simulink model "Version_Nov_21"  (R2022a)
settings: Solver=FixedStepAuto  StartTime=0.0  StopTime=60  FixedStep=1e-3  RelTol=1e-3  EnableMultiTasking=on
undefined symbols (not defined in the file): D10, D11, D12, D13, D2, D3, D4, D5, D6, D7, D8, D9, PTA0, PTA1, PTA2, PTB23, PTB9, PTC2, PTC3, PTC4, PTD0, PTD1, PTD2, PTD3
libraries: frdmk64flib x13
settings Model: ExtModeTrigDuration=5  Creator=ethan  LastModifiedBy=ethan
settings OptimizationCC: EnhancedBackFolding=on  PassReuseOutputArgsAs=Individual arguments  ZeroExternalMemoryAtStartup=off  ZeroInternalMemoryAtStartup=off  MaxStackSize=64  OptimizeBlockOrder=speed  DifferentSizesBufferReuse=on  OptimizationCustomize=off  EfficientTunableParamExpr=on
settings DebuggingCC: ParameterTunabilityLossMsg=error
settings HardwareCC: ProdBitPerPointer=32  ProdBitPerSizeT=32  ProdBitPerPtrDiffT=32  ProdLargestAtomicInteger=Long  ProdLargestAtomicFloat=Double  ProdWordSize=32  ProdHWDeviceType=ARM Compatible->ARM Cortex
settings SFSimCC: MATLABDynamicMemAlloc=off
settings RTWCC: SystemTargetFile=ert.tlc  HardwareBoard=NXP FRDM-K64F  TLCOptions="-aInlineSetEventsForThisBaseRateFcn=TLC_FALSE -aSuppressMultiTaskScheduler=TLC_FALSE  -aRateBasedStepFcn=0"  TemplateMakefile=ert_default_tmf  Toolchain=GNU Tools for ARM Embedded Processors
settings CodeAppCC: ForceParamTrailComments=on  IgnoreCustomStorageClasses=off  OperatorAnnotations=on  SimulinkDataObjDesc=on  SFDataObjDesc=on  InsertBlockDesc=on
settings ERTTargetCC: ExtModeTransport=4  ExtModeMexFile=sendToCommService

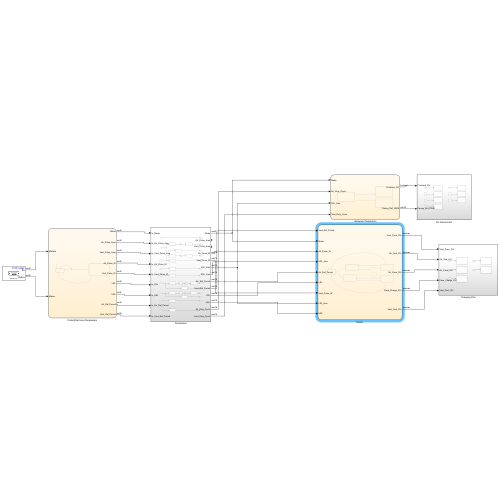
[thumbnail: Simulink's stored preview of the top-level diagram]
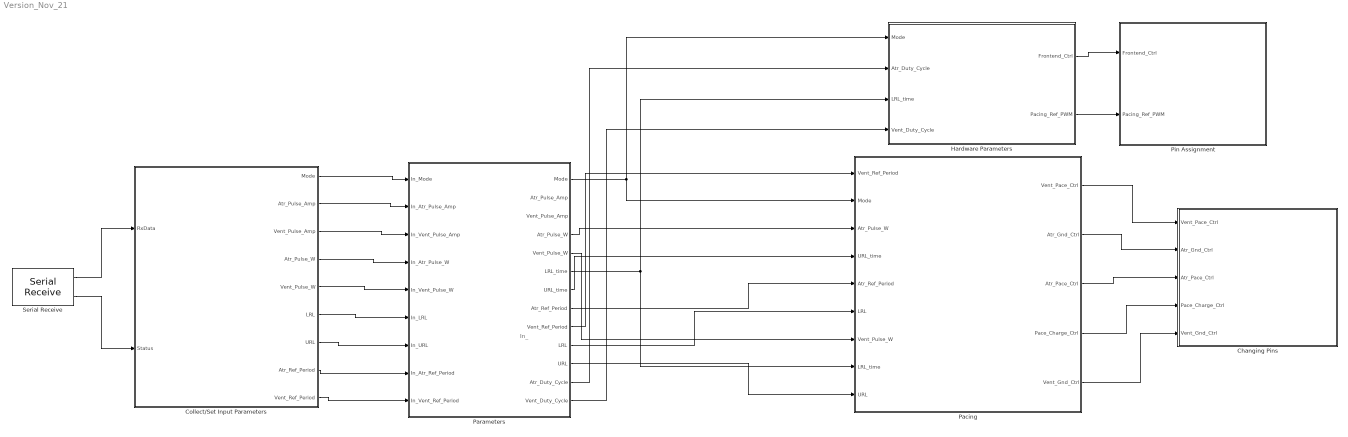
== system Version_Nov_21 ==
  note: In_
  Changing Pins : Subsystem
  Collect/Set Input Parameters : Stateflow chart  TreatAsAtomicUnit=on
      settings: PortSchema="{\"entries\":[{\"content\":{\"sides\":[{\"content\":{\"connectorIds\":[\"In1\",\"In2\"]},\"type\":\"ConnectorPlacement.EquallySpacedRectSide\",\"uuid\":\"dc51e4f5-5341-418f-80a9-38d3dc8e9b6e\"},{\"content\":{\"connectorIds\":[\"Out1\",\"Out3\",\"Out6\",\"Out2\",\"Out7\",\"Out9\",\"Out5\",\"Out4\",\"Out8\"],\"side\":\"RIGHT\"},\"type\":\"ConnectorPlacement.EquallySpacedRectSide\",\"uuid\":\"313c6298-b0b7-4ff0-85ba-dbaa1c18177a\"},{\"content\":{\"connectorIds\":[],\"side\":\"TOP\"},\"type\":\"ConnectorPlacement.EquallySpacedRectSide\",\"uuid\":\"6f377806-6de9-4b84-8111-50855010f7f2\"}]},\"type\":\"ConnectorPlacement.EquallySpacedConnector\",\"uuid\":\"8b0403f6-9322-46f9-82a4-778a28822a3d\"}],\"packageUris\":[\"http://schema.mathworks.com/mf0/Connector/R2020b\"],\"version\":\"1.0\"}"
  Hardware Parameters : Stateflow chart  TreatAsAtomicUnit=on
  Pacing : Stateflow chart  TreatAsAtomicUnit=on
      settings: PortSchema="{\"entries\":[{\"content\":{\"sides\":[{\"content\":{\"connectorIds\":[\"In9\",\"In1\",\"In3\",\"In6\",\"In7\",\"In8\",\"In4\",\"In5\",\"In2\"]},\"type\":\"ConnectorPlacement.EquallySpacedRectSide\",\"uuid\":\"cbd26b3d-27cb-4744-9a6d-2e29f16e2c2e\"},{\"content\":{\"connectorIds\":[\"Out1\",\"Out2\",\"Out3\",\"Out4\",\"Out5\"],\"side\":\"RIGHT\"},\"type\":\"ConnectorPlacement.EquallySpacedRectSide\",\"uuid\":\"25c89074-e17e-4898-a31a-c42a3e343a2e\"},{\"content\":{\"connectorIds\":[],\"side\":\"TOP\"},\"type\":\"ConnectorPlacement.EquallySpacedRectSide\",\"uuid\":\"e4014b57-3770-4bf4-bd9b-5c9114757f0a\"}]},\"type\":\"ConnectorPlacement.EquallySpacedConnector\",\"uuid\":\"9ef350bf-8d26-4971-b7d1-0d0774d6b5a5\"}],\"packageUris\":[\"http://schema.mathworks.com/mf0/Connector/R2020b\"],\"version\":\"1.0\"}"
  Parameters : Subsystem
  Pin Assignment : Subsystem
  Serial Receive : frdmk64flib/Serial Receive  SCIModule=0  Baudrate=uint32(9600)  Parity=None  StopBits=1  HardwareFlowControl=None  ByteOrder=LittleEndian  DataType=uint8  DataLength=10  BlockingMode=off  OutputStatus=on  SampleTime=-1
  wires:
  Serial Receive/1 -> Collect/Set Input Parameters/1(RxData)
  Serial Receive/2 -> Collect/Set Input Parameters/2(Status)
  Collect/Set Input Parameters/1(Mode) -> Parameters/1(In_Mode)
  Collect/Set Input Parameters/3(Atr_Pulse_Amp) -> Parameters/2(In_Atr_Pulse_Amp)
  Collect/Set Input Parameters/6(Vent_Pulse_Amp) -> Parameters/3(In_Vent_Pulse_Amp)
  Collect/Set Input Parameters/4(Atr_Ref_Period) -> Parameters/8(In_Atr_Ref_Period)
  Collect/Set Input Parameters/5(URL) -> Parameters/7(In_URL)
  Collect/Set Input Parameters/9(LRL) -> Parameters/6(In_LRL)
  Collect/Set Input Parameters/8(Vent_Ref_Period) -> Parameters/9(In_Vent_Ref_Period)
  Collect/Set Input Parameters/2(Atr_Pulse_W) -> Parameters/4(In_Atr_Pulse_W)
  Pacing/1(Vent_Pace_Ctrl) -> Changing Pins/1(Vent_Pace_Ctrl)
  Pacing/2(Atr_Gnd_Ctrl) -> Changing Pins/2(Atr_Gnd_Ctrl)
  Pacing/3(Atr_Pace_Ctrl) -> Changing Pins/3(Atr_Pace_Ctrl)
  Pacing/4(Pace_Charge_Ctrl) -> Changing Pins/4(Pace_Charge_Ctrl)
  Pacing/5(Vent_Gnd_Ctrl) -> Changing Pins/5(Vent_Gnd_Ctrl)
  Collect/Set Input Parameters/7(Vent_Pulse_W) -> Parameters/5(In_Vent_Pulse_W)
  Parameters/1(Mode) -> Hardware Parameters/1(Mode), Pacing/1(Mode)
  Parameters/4(Atr_Pulse_W) -> Pacing/3(Atr_Pulse_W)
  Parameters/5(Vent_Pulse_W) -> Pacing/4(Vent_Pulse_W)
  Parameters/6(LRL_time) -> Hardware Parameters/3(LRL_time), Pacing/5(LRL_time)
  Parameters/7(URL_time) -> Pacing/6(URL_time)
  Parameters/8(Atr_Ref_Period) -> Pacing/7(Atr_Ref_Period)
  Parameters/9(Vent_Ref_Period) -> Pacing/9(Vent_Ref_Period)
  Parameters/10(LRL) -> Pacing/8(LRL)
  Parameters/11(URL) -> Pacing/2(URL)
  Parameters/12(Atr_Duty_Cycle) -> Hardware Parameters/2(Atr_Duty_Cycle)
  Parameters/13(Vent_Duty_Cycle) -> Hardware Parameters/4(Vent_Duty_Cycle)
  Hardware Parameters/1(Frontend_Ctrl) -> Pin Assignment/1(Frontend_Ctrl)
  Hardware Parameters/2(Pacing_Ref_PWM) -> Pin Assignment/2(Pacing_Ref_PWM)

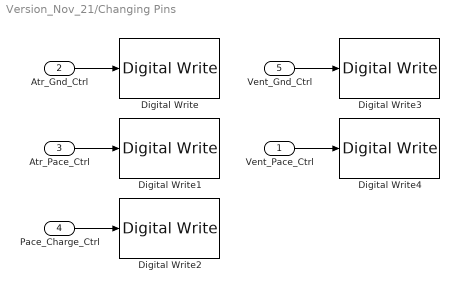
== system Version_Nov_21/Changing Pins ==
  Vent_Pace_Ctrl : Inport
  Atr_Gnd_Ctrl : Inport  Port=2
  Atr_Pace_Ctrl : Inport  Port=3
  Pace_Charge_Ctrl : Inport  Port=4
  Vent_Gnd_Ctrl : Inport  Port=5
  Digital Write : frdmk64flib/Digital Write  Whichpin=PTD2 (D11)
  Digital Write1 : frdmk64flib/Digital Write  Whichpin=PTA0 (D8)
  Digital Write2 : frdmk64flib/Digital Write  Whichpin=PTB9 (D2)
  Digital Write3 : frdmk64flib/Digital Write  Whichpin=PTD3 (D12)
  Digital Write4 : frdmk64flib/Digital Write  Whichpin=PTC4 (D9)
  wires:
  Atr_Gnd_Ctrl/1 -> Digital Write/1
  Atr_Pace_Ctrl/1 -> Digital Write1/1
  Pace_Charge_Ctrl/1 -> Digital Write2/1
  Vent_Gnd_Ctrl/1 -> Digital Write3/1
  Vent_Pace_Ctrl/1 -> Digital Write4/1

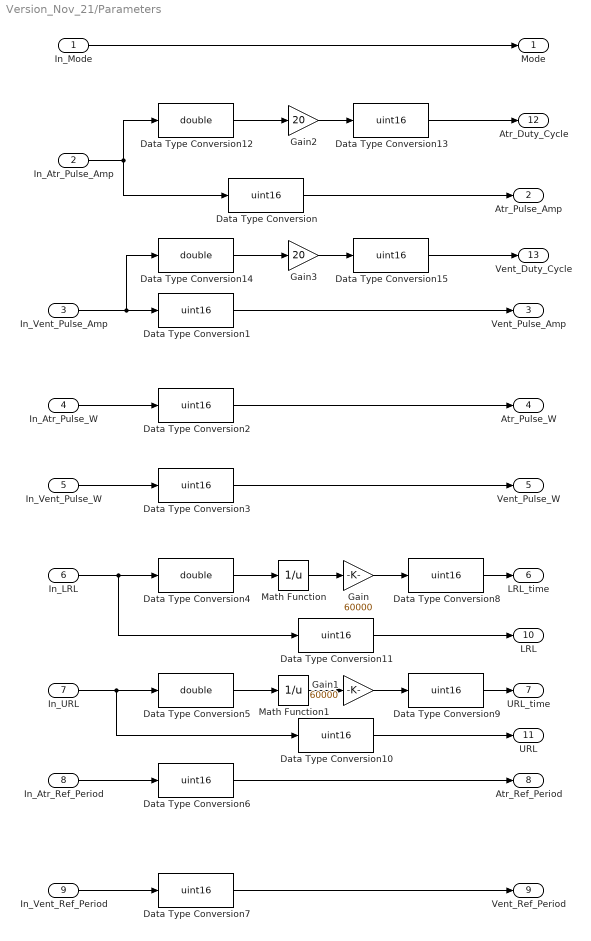
== system Version_Nov_21/Parameters ==
  In_Mode : Inport
  In_Atr_Pulse_Amp : Inport  Port=2
  In_Vent_Pulse_Amp : Inport  Port=3
  In_Atr_Pulse_W : Inport  Port=4
  In_Vent_Pulse_W : Inport  Port=5
  In_LRL : Inport  Port=6
  In_URL : Inport  Port=7
  In_Atr_Ref_Period : Inport  Port=8
  In_Vent_Ref_Period : Inport  Port=9
  Data Type Conversion{,1..3,6..11,13,15} (12 alike) : DataTypeConversion  OutDataTypeStr=uint16  SaturateOnIntegerOverflow=off  RndMeth=Floor
  Data Type Conversion{4..5,12,14} (4 alike) : DataTypeConversion  OutDataTypeStr=double  SaturateOnIntegerOverflow=off  RndMeth=Floor
  Gain : Gain  Gain=60000
  Gain1 : Gain  Gain=60000
  Gain2 : Gain  Gain=20
  Gain3 : Gain  Gain=20
  Math Function : Math  Operator=reciprocal
  Math Function1 : Math  Operator=reciprocal
  Mode : Outport
  Atr_Pulse_Amp : Outport  Port=2
  Vent_Pulse_Amp : Outport  Port=3
  Atr_Pulse_W : Outport  Port=4
  Vent_Pulse_W : Outport  Port=5
  LRL_time : Outport  Port=6
  URL_time : Outport  Port=7
  Atr_Ref_Period : Outport  Port=8
  Vent_Ref_Period : Outport  Port=9
  LRL : Outport  Port=10
  URL : Outport  Port=11
  Atr_Duty_Cycle : Outport  Port=12
  Vent_Duty_Cycle : Outport  Port=13
  wires:
  In_Mode/1 -> Mode/1
  Data Type Conversion/1 -> Atr_Pulse_Amp/1
  In_Vent_Pulse_Amp/1 -> Data Type Conversion14/1, Data Type Conversion1/1
  Data Type Conversion1/1 -> Vent_Pulse_Amp/1
  In_Atr_Pulse_W/1 -> Data Type Conversion2/1
  Data Type Conversion2/1 -> Atr_Pulse_W/1
  In_Vent_Pulse_W/1 -> Data Type Conversion3/1
  Data Type Conversion3/1 -> Vent_Pulse_W/1
  In_LRL/1 -> Data Type Conversion11/1, Data Type Conversion4/1
  Data Type Conversion4/1 -> Math Function/1
  Math Function/1 -> Gain/1
  Gain/1 -> Data Type Conversion8/1
  In_URL/1 -> Data Type Conversion10/1, Data Type Conversion5/1
  Data Type Conversion5/1 -> Math Function1/1
  Math Function1/1 -> Gain1/1
  Gain1/1 -> Data Type Conversion9/1
  In_Vent_Ref_Period/1 -> Data Type Conversion7/1
  Data Type Conversion7/1 -> Vent_Ref_Period/1
  In_Atr_Ref_Period/1 -> Data Type Conversion6/1
  Data Type Conversion6/1 -> Atr_Ref_Period/1
  Data Type Conversion8/1 -> LRL_time/1
  Data Type Conversion9/1 -> URL_time/1
  Data Type Conversion10/1 -> URL/1
  Data Type Conversion11/1 -> LRL/1
  In_Atr_Pulse_Amp/1 -> Data Type Conversion12/1, Data Type Conversion/1
  Gain2/1 -> Data Type Conversion13/1
  Data Type Conversion13/1 -> Atr_Duty_Cycle/1
  Data Type Conversion12/1 -> Gain2/1
  Data Type Conversion15/1 -> Vent_Duty_Cycle/1
  Gain3/1 -> Data Type Conversion15/1
  Data Type Conversion14/1 -> Gain3/1

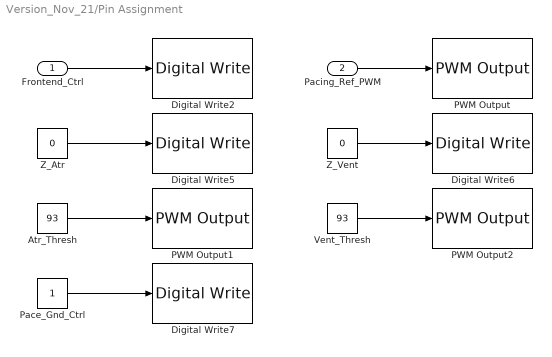
== system Version_Nov_21/Pin Assignment ==
  Frontend_Ctrl : Inport
  Pacing_Ref_PWM : Inport  Port=2
  Atr_Thresh : Constant  Value=93
  Digital Write2 : frdmk64flib/Digital Write  Whichpin=PTD1 (D13)
  Digital Write5 : frdmk64flib/Digital Write  Whichpin=PTB23 (D4)
  Digital Write6 : frdmk64flib/Digital Write  Whichpin=PTC3 (D7)
  Digital Write7 : frdmk64flib/Digital Write  Whichpin=PTD0 (D10)
  PWM Output : frdmk64flib/PWM Output  Whichpin=PTA2 (D5)  InitialFrequency=2000  InitialDutyCycle=0
  PWM Output1 : frdmk64flib/PWM Output  Whichpin=PTC2 (D6)  InitialFrequency=2000  InitialDutyCycle=0
  PWM Output2 : frdmk64flib/PWM Output  Whichpin=PTA1 (D3)  InitialFrequency=2000  InitialDutyCycle=0
  Pace_Gnd_Ctrl : Constant
  Vent_Thresh : Constant  Value=93
  Z_Atr : Constant  Value=0
  Z_Vent : Constant  Value=0
  wires:
  Frontend_Ctrl/1 -> Digital Write2/1
  Z_Atr/1 -> Digital Write5/1
  Z_Vent/1 -> Digital Write6/1
  Vent_Thresh/1 -> PWM Output2/1
  Atr_Thresh/1 -> PWM Output1/1
  Pace_Gnd_Ctrl/1 -> Digital Write7/1
  Pacing_Ref_PWM/1 -> PWM Output/1

== stateflow chart Version_Nov_21/Pacing ==
  state VOO_Charge
    entry:
    Vent_Pace_Ctrl = false;
    Vent_Gnd_Ctrl = true;
    Atr_Gnd_Ctrl = false;
    Atr_Pace_Ctrl = false;
    Pace_Charge_Ctrl = true;
  state VOO_Discharge
    entry:
    Vent_Pace_Ctrl = true;
    Vent_Gnd_Ctrl = false;
    Pace_Charge_Ctrl = false;
  state Initial_State
    entry:
  state Light [commented out]
    entry:
    Green = true;
  state AOO_Charge
    entry:
    Atr_Gnd_Ctrl = true;
    Atr_Pace_Ctrl = false;
    Vent_Pace_Ctrl = false;
    Vent_Gnd_Ctrl = false;
    Pace_Charge_Ctrl = true;
  state AOO_Discharge
    entry:
    Atr_Gnd_Ctrl = false;
    Atr_Pace_Ctrl = true;
    Pace_Charge_Ctrl = false;
  VOO_Discharge -> Initial_State [order 1] : [Mode ~= 1]
  VOO_Discharge -> VOO_Charge [order 2] : after(Vent_Pulse_W,msec)
  (junction 66) -> VOO_Discharge : [after((LRL_time)-Vent_Pulse_W,msec)]
  (default) -> Initial_State
  Initial_State -> VOO_Charge [order 1] : [Mode == 1]
  VOO_Charge -> (junction 66)
  Light -> (junction 66) [commented out]
  (junction 66) -> Light [commented out] : [LRL-Vent_Pulse_W == 980]
  Initial_State -> AOO_Charge [order 2] : [Mode == 2]
  AOO_Discharge -> Initial_State [order 1] : [Mode ~= 2]
  AOO_Discharge -> AOO_Charge [order 2] : after(Atr_Pulse_W,msec)
  AOO_Charge -> AOO_Discharge : after(LRL_time-Atr_Pulse_W,msec)
  data: Mode input; URL input; Atr_Pulse_W input uint16; Vent_Pulse_W input uint16; LRL_time input uint16; URL_time input; Atr_Ref_Period input; LRL input uint16; Vent_Ref_Period input; Vent_Pace_Ctrl output boolean; Atr_Gnd_Ctrl output boolean; Atr_Pace_Ctrl output boolean; Pace_Charge_Ctrl output; Vent_Gnd_Ctrl output; Cur_Mode local

== stateflow chart Version_Nov_21/Hardware Parameters ==
  state Set_Parameters_VOO_VOOR
    entry:
    Pacing_Ref_PWM = Vent_Duty_Cycle;
    Frontend_Ctrl = false;
  state Initialize_Variables
    entry:
  state Set_Parameters_AOO_AOOR
    entry:
    Pacing_Ref_PWM = Atr_Duty_Cycle;
    Frontend_Ctrl = false;
  (default) -> Initialize_Variables
  Initialize_Variables -> Set_Parameters_VOO_VOOR [order 1] : [Mode == 1 || Mode == 5]
  Initialize_Variables -> Set_Parameters_AOO_AOOR [order 2] : [Mode == 2 || Mode == 6]
  data: Mode input; Atr_Duty_Cycle input uint16; LRL_time input; Vent_Duty_Cycle input uint16; Frontend_Ctrl output; Pacing_Ref_PWM output uint16

== stateflow chart Version_Nov_21/Collect//Set Input Parameters ==
  state Input_Parameters
    entry:
    Mode = RxData(2);
    LRL = RxData(3);
    URL = RxData(4);
    Vent_Pulse_W = RxData(5);
    Atr_Pulse_W = RxData(6);
    Vent_Pulse_Amp = RxData(7);
    Atr_Pulse_Amp = RxData(8);
    Vent_Ref_Period = RxData(9);
    Atr_Ref_Period = RxData(10);
  state Wait_For_Transmission
  (default) -> Wait_For_Transmission
  (junction 16) -> Wait_For_Transmission [order 2]
  Wait_For_Transmission -> (junction 16) : [Status == 0]
  (junction 16) -> Input_Parameters [order 1] : [RxData(1) == hex2dec('10')]
  Input_Parameters -> Wait_For_Transmission
  data: RxData input; Status input; Mode output; Atr_Pulse_W output uint8; Atr_Pulse_Amp output uint8; Atr_Ref_Period output uint8; URL output uint8; Vent_Pulse_Amp output uint8; Vent_Pulse_W output uint8; Vent_Ref_Period output uint8; LRL output uint8
